simulink model "uz_park_transformation"  (R2021a)
settings: Solver=FixedStepDiscrete  StartTime=0.0  StopTime=0.01  RelTol=1e-3
values from neighbouring files (symbols this model uses):
  freq_Hz = 300    [uz_park_transformation_init.m]
  t_ADC = 1/f_ADC    (= 1e-05)    [uz_park_transformation_init.m]
libraries: simulink x1, hdlsllib x1
settings Model: DataTypeOverride=Off  Creator=micha  LastModifiedBy=micha
settings SolverCC: AlgebraicLoopSolver=TrustRegion
settings DataIOCC: LimitDataPoints=on  SaveOutput=off  SaveTime=off
settings OptimizationCC: BlockReduction=off  ConditionallyExecuteInputs=off  DefaultParameterBehavior=Inlined  LifeSpan=inf
settings DebuggingCC: AlgebraicLoopMsg=error  SingleTaskRateTransMsg=error  AllowSymbolicDim=off  StrictBusMsg=ErrorOnBusTreatedAsVector  SFUnexpectedBacktrackingDiag=warning  SFNoUnconditionalDefaultTransitionDiag=warning  SFExecutionAtInitializationDiag=none  SFMachineParentedDataDiag=warning  ArithmeticOperatorsInVariantConditions=warning
settings HardwareCC: ProdBitPerPointer=32  ProdBitPerSizeT=32  ProdBitPerPtrDiffT=32  ProdLargestAtomicFloat=None  ProdIntDivRoundTo=Undefined  ProdEndianess=Unspecified  ProdWordSize=32  ProdHWDeviceType=ASIC/FPGA->ASIC/FPGA  ProdEqTarget=off
settings SFSimCC: SimUseLocalCustomCode=off  CustomCodeUndefinedFunction=UseInterfaceOnly
settings RTWCC: RTWUseLocalCustomCode=off
settings CodeAppCC: StateflowObjectComments=on
settings GRTTargetCC: TargetLangStandard=C89/C90 (ANSI)
settings ConfigComp: CovScope=ReferencedModels  CovMetricSettings=dw  CovSaveCumulativeToWorkspaceVar=on  CovSaveSingleToWorkspaceVar=on  CovExternalEMLEnable=off  CovSFcnEnable=off

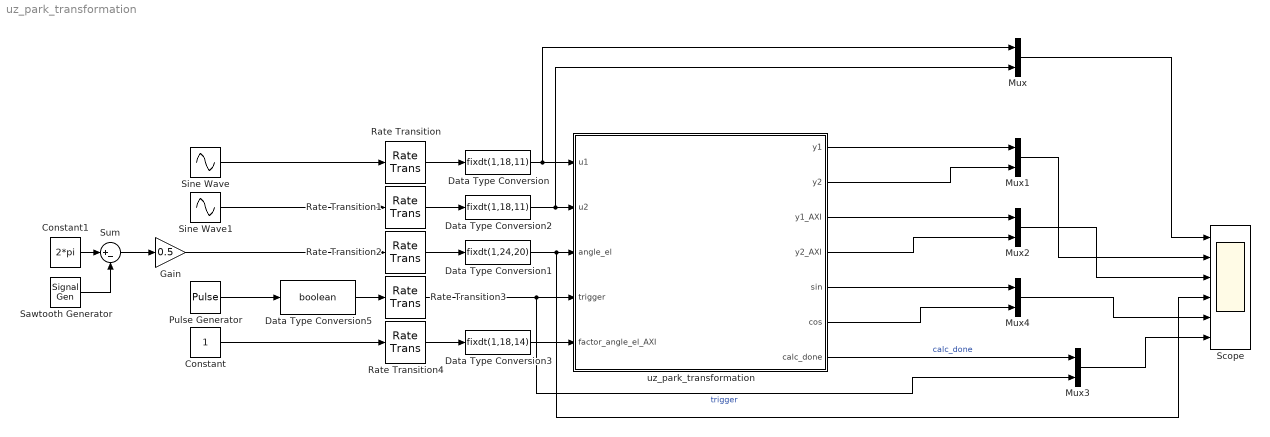
== system uz_park_transformation ==
  Constant : Constant
  Constant1 : Constant  Value=2*pi
  Data Type Conversion : DataTypeConversion  OutDataTypeStr=fixdt(1,18,11)
  Data Type Conversion1 : DataTypeConversion  OutDataTypeStr=fixdt(1,24,20)
  Data Type Conversion2 : DataTypeConversion  OutDataTypeStr=fixdt(1,18,11)
  Data Type Conversion3 : DataTypeConversion  OutDataTypeStr=fixdt(1,18,14)
  Data Type Conversion5 : DataTypeConversion  OutDataTypeStr=boolean
  Gain : Gain  Gain=0.5
  Mux{,1..4} (5 alike) : Mux  Inputs=2
  Pulse Generator : DiscretePulseGenerator  PulseType=Time based  Period=t_ADC  PulseWidth=5
  Rate Transition{,1..4} (5 alike) : RateTransition  OutPortSampleTime=t_clock
  Sawtooth Generator : SignalGenerator  WaveForm=sawtooth  Amplitude=2*pi  Frequency=2*pi*freq_Hz  Units=rad/sec
  Scope : Scope  NumInputPorts=6
  Sine Wave : Sin  Frequency=2*pi*freq_Hz  SampleTime=0
  Sine Wave1 : Sin  Frequency=2*pi*freq_Hz  Phase=-pi/2  SampleTime=0
  Sum : Sum  Inputs=|+-
  uz_park_transformation : Subsystem  TreatAsAtomicUnit=on
  wires:
  uz_park_transformation/1(y1) -> Mux1/1
  Rate Transition/1 -> Data Type Conversion/1
  Rate Transition1/1 -> Data Type Conversion2/1
  Rate Transition2/1 -> Data Type Conversion1/1
  Rate Transition3/1 -> Mux3/2, uz_park_transformation/4(trigger)  "trigger"
  Rate Transition4/1 -> Data Type Conversion3/1
  Constant/1 -> Rate Transition4/1
  Pulse Generator/1 -> Data Type Conversion5/1
  Data Type Conversion5/1 -> Rate Transition3/1
  uz_park_transformation/2(y2) -> Mux1/2
  Sine Wave/1 -> Rate Transition/1
  Sine Wave1/1 -> Rate Transition1/1
  Gain/1 -> Rate Transition2/1
  Sawtooth Generator/1 -> Sum/2
  Constant1/1 -> Sum/1
  Sum/1 -> Gain/1
  Data Type Conversion/1 -> Mux/1, uz_park_transformation/1(u1)
  Data Type Conversion1/1 -> Scope/4, uz_park_transformation/3(angle_el)
  Data Type Conversion2/1 -> Mux/2, uz_park_transformation/2(u2)
  Data Type Conversion3/1 -> uz_park_transformation/5(factor_angle_el_AXI)
  Mux/1 -> Scope/1
  Mux1/1 -> Scope/2
  uz_park_transformation/3(y1_AXI) -> Mux2/1
  uz_park_transformation/4(y2_AXI) -> Mux2/2
  Mux2/1 -> Scope/3
  uz_park_transformation/7(calc_done) -> Mux3/1  "calc_done"
  Mux3/1 -> Scope/6
  uz_park_transformation/5(sin) -> Mux4/1
  uz_park_transformation/6(cos) -> Mux4/2
  Mux4/1 -> Scope/5

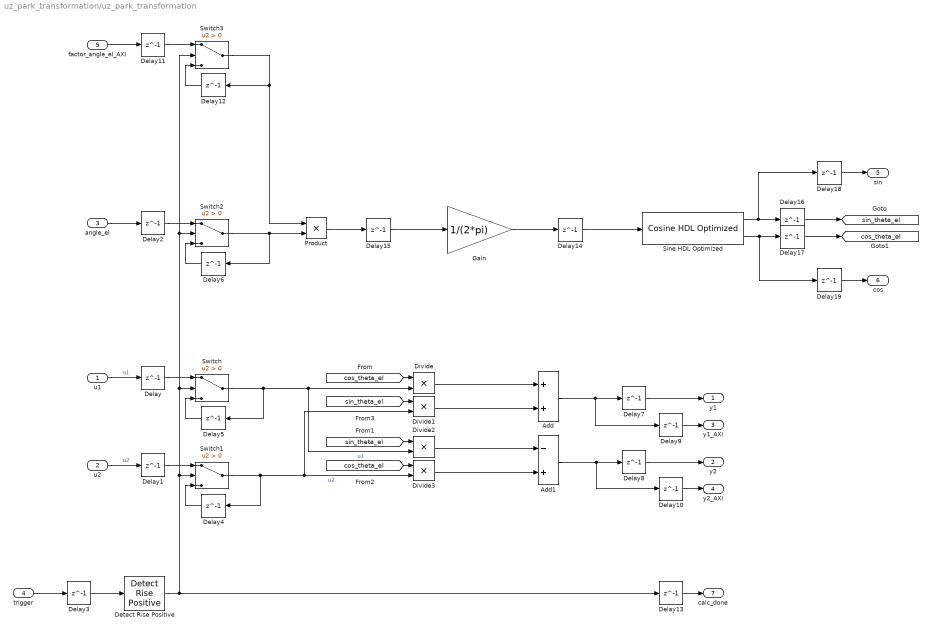
== system uz_park_transformation/uz_park_transformation ==
  u1 : Inport
  u2 : Inport  Port=2
  angle_el : Inport  Port=3
  trigger : Inport  Port=4
  factor_angle_el_AXI : Inport  Port=5
  Add : Sum  OutDataTypeStr=fixdt(1,27,16)
  Add1 : Sum  Inputs=-+  OutDataTypeStr=fixdt(1,27,16)
  Delay{,1..19} (20 alike) : Delay  DelayLength=1
  Detect Rise Positive : simulink/Logic and Bit Operations/Detect Rise Positive  vinit=0  OutDataTypeStr=boolean
  Divide{,1..3} (4 alike) : Product  Inputs=**  OutDataTypeStr=fixdt(1,27,16)
  Gain : Gain  Gain=1/(2*pi)  OutDataTypeStr=fixdt(1,18,16)
  Product : Product  OutDataTypeStr=fixdt(1,18,14)
  Sine HDL Optimized : hdlsllib/Lookup Tables/Cosine HDL Optimized  OutputFormula=sin(2*pi*u) and cos(2*pi*u)  NumDataPoints=256  TableDataTypeStr=fixdt(0,17,16)  SimulateLUTROMDelay=off
      settings: SourceProductBaseCode=SL
  Switch{,1..3} (4 alike) : Switch  Criteria=u2 > Threshold
  y1 : Outport  VectorParamsAs1DForOutWhenUnconnected=off
  y2 : Outport  Port=2  VectorParamsAs1DForOutWhenUnconnected=off
  y1_AXI : Outport  Port=3  VectorParamsAs1DForOutWhenUnconnected=off
  y2_AXI : Outport  Port=4  VectorParamsAs1DForOutWhenUnconnected=off
  sin : Outport  Port=5  VectorParamsAs1DForOutWhenUnconnected=off
  cos : Outport  Port=6  VectorParamsAs1DForOutWhenUnconnected=off
  calc_done : Outport  Port=7  VectorParamsAs1DForOutWhenUnconnected=off
  tag scope: cos_theta_el=global, sin_theta_el=global
  wires:
  Switch1/1 -> Delay4/1, Divide1/2, Divide3/2  "u2"
  Divide2/1 -> Add1/1
  Divide3/1 -> Add1/2
  [cos_theta_el] -> Divide3/1
  Switch/1 -> Divide2/2, Divide/2, Delay5/1  "u1"
  [sin_theta_el] -> Divide2/1
  Divide1/1 -> Add/2
  [cos_theta_el] -> Divide/1
  [sin_theta_el] -> Divide1/1
  Add/1 -> Delay9/1, Delay7/1
  Add1/1 -> Delay10/1, Delay8/1
  Divide/1 -> Add/1
  angle_el/1 -> Delay2/1
  Sine HDL Optimized/2 -> Delay19/1, Delay17/1
  Sine HDL Optimized/1 -> Delay18/1, Delay16/1
  Gain/1 -> Delay14/1
  u1/1 -> Delay/1  "u1"
  u2/1 -> Delay1/1  "u2"
  Delay/1 -> Switch/1
  Delay1/1 -> Switch1/1
  Delay2/1 -> Switch2/1
  trigger/1 -> Delay3/1
  Delay4/1 -> Switch1/3
  Delay5/1 -> Switch/3
  Delay6/1 -> Switch2/3
  Delay7/1 -> y1/1
  Delay8/1 -> y2/1
  Delay9/1 -> y1_AXI/1
  Delay10/1 -> y2_AXI/1
  Switch2/1 -> Product/2, Delay6/1
  Switch3/1 -> Product/1, Delay12/1
  factor_angle_el_AXI/1 -> Delay11/1
  Detect Rise Positive/1 -> Delay13/1, Switch1/2, Switch/2, Switch3/2, Switch2/2
  Delay12/1 -> Switch3/3
  Delay11/1 -> Switch3/1
  Product/1 -> Delay15/1
  Delay3/1 -> Detect Rise Positive/1
  Delay13/1 -> calc_done/1
  Delay15/1 -> Gain/1
  Delay14/1 -> Sine HDL Optimized/1
  Delay16/1 -> [sin_theta_el]
  Delay17/1 -> [cos_theta_el]
  Delay18/1 -> sin/1
  Delay19/1 -> cos/1
